simulink model "prob3"  (R2019a)
settings: Solver=VariableStepAuto  StartTime=0.0  StopTime=10.0  RelTol=1e-3
values from neighbouring files (symbols this model uses):
  accBias = 1E-3 * g    [prob3main.m]
  C1 = 3/tau    [prob3main.m]
  C2 = 2*schuler^2 + 3/tau/tau    [prob3main.m]
  C3 = 1/(tau^3)    [prob3main.m]
  C4 = 0    [prob3main.m]
  schuler = sqrt(g/R)    [prob3main.m]
  tauH = 1000    [prob3main.m]
undefined symbols (not defined in the file or in its folder): varH
settings Model: Creator=hyunwoong  LastModifiedBy=hyunwoong

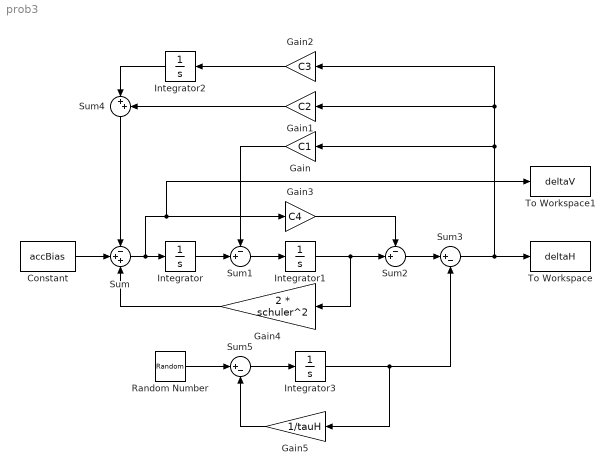
== system prob3 ==
  Constant : Constant  Value=accBias
  Gain : Gain  Gain=C1
  Gain1 : Gain  Gain=C2
  Gain2 : Gain  Gain=C3
  Gain3 : Gain  Gain=C4
  Gain4 : Gain  Gain=2 * schuler^2
  Gain5 : Gain  Gain=1/tauH
  Integrator{,1..3} (4 alike) : Integrator
  Random Number : RandomNumber  Variance=varH  SampleTime=0.1
  Sum : Sum  Inputs=-++
  Sum1 : Sum  Inputs=-+|
  Sum2 : Sum  Inputs=-+|
  Sum3 : Sum  Inputs=|+-
  Sum4 : Sum  Inputs=|++
  Sum5 : Sum  Inputs=|+-
  To Workspace : ToWorkspace  VariableName=deltaH  SaveFormat=Timeseries  SampleTime=-1
  To Workspace1 : ToWorkspace  VariableName=deltaV  SaveFormat=Timeseries  SampleTime=-1
  wires:
  Constant/1 -> Sum/2
  Sum/1 -> To Workspace1/1, Gain3/1, Integrator/1
  Integrator/1 -> Sum1/2
  Sum1/1 -> Integrator1/1
  Integrator1/1 -> Gain4/1, Sum2/2
  Gain3/1 -> Sum2/1
  Gain/1 -> Sum1/1
  Gain2/1 -> Integrator2/1
  Gain1/1 -> Sum4/2
  Integrator2/1 -> Sum4/1
  Sum4/1 -> Sum/1
  Sum3/1 -> To Workspace/1, Gain1/1, Gain2/1, Gain/1
  Sum2/1 -> Sum3/1
  Gain4/1 -> Sum/3
  Gain5/1 -> Sum5/2
  Integrator3/1 -> Gain5/1, Sum3/2
  Sum5/1 -> Integrator3/1
  Random Number/1 -> Sum5/1
